simulink model "Z3"  (R2016b)
settings: Solver=VariableStepAuto  StartTime=0.0  StopTime=2  RelTol=1e-3
values from neighbouring files (symbols this model uses):
  x0 = [0.1 0.1 0.1]    [z3.m]    (also in z6.m = [-1 2 1]; z7.m = [0 0 0]; z8.m = [-1 2 1])
settings Model: Creator=E7440  LastModifiedBy=E7440

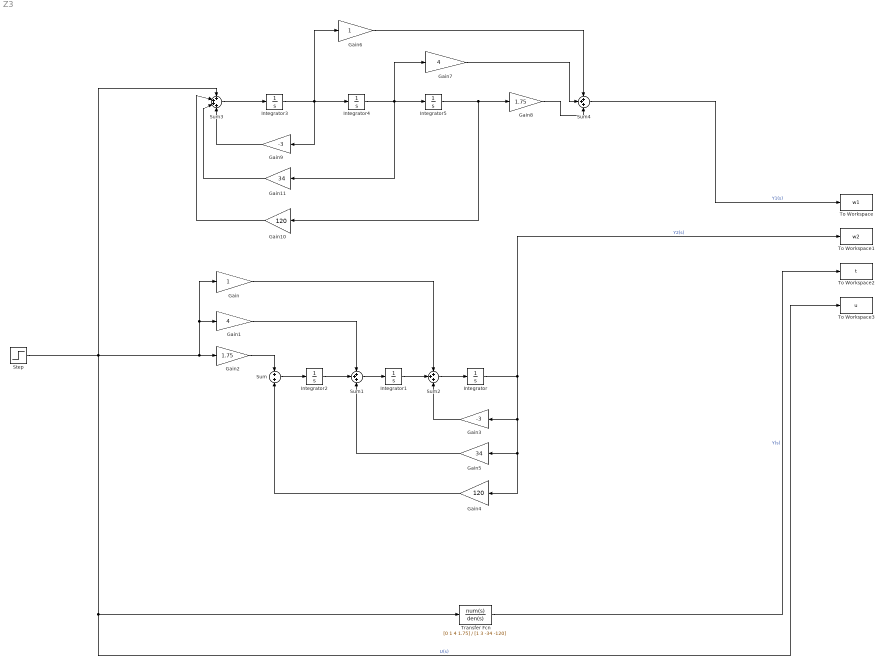
== system Z3 ==
  Gain : Gain
  Gain1 : Gain  Gain=4
  Gain10 : Gain  Gain=120
  Gain11 : Gain  Gain=34
  Gain2 : Gain  Gain=1.75
  Gain3 : Gain  Gain=-3
  Gain4 : Gain  Gain=120
  Gain5 : Gain  Gain=34
  Gain6 : Gain
  Gain7 : Gain  Gain=4
  Gain8 : Gain  Gain=1.75
  Gain9 : Gain  Gain=-3
  Integrator : Integrator  InitialCondition=x0(3)
  Integrator1 : Integrator  InitialCondition=x0(2)
  Integrator2 : Integrator  InitialCondition=x0(1)
  Integrator3 : Integrator  InitialCondition=x0(1)
  Integrator4 : Integrator  InitialCondition=x0(2)
  Integrator5 : Integrator  InitialCondition=x0(3)
  Step : Step  SampleTime=0
  Sum : Sum
  Sum1 : Sum  Inputs=+++
  Sum2 : Sum  Inputs=+++
  Sum3 : Sum  Inputs=++++
  Sum4 : Sum  Inputs=+++
  To Workspace : ToWorkspace  VariableName=w1  SaveFormat=Timeseries  SampleTime=-1
  To Workspace1 : ToWorkspace  VariableName=w2  SaveFormat=Timeseries  SampleTime=-1
  To Workspace2 : ToWorkspace  VariableName=t  SaveFormat=Timeseries  SampleTime=-1
  To Workspace3 : ToWorkspace  VariableName=u  SaveFormat=Timeseries  SampleTime=-1
  Transfer Fcn : TransferFcn  Numerator=[0 1 4 1.75]  Denominator=[1 3 -34 -120]
  wires:
  Sum/1 -> Integrator2/1
  Gain3/1 -> Sum2/3
  Integrator/1 -> To Workspace1/1, Gain3/1, Gain5/1, Gain4/1  "Y2(s)"
  Gain2/1 -> Sum/1
  Integrator1/1 -> Sum2/2
  Sum2/1 -> Integrator/1
  Integrator2/1 -> Sum1/2
  Sum1/1 -> Integrator1/1
  Gain5/1 -> Sum1/3
  Gain4/1 -> Sum/2
  Gain/1 -> Sum2/1
  Gain1/1 -> Sum1/1
  Step/1 -> To Workspace3/1, Transfer Fcn/1, Sum3/1, Gain/1, Gain1/1, Gain2/1  "U(s)"
  Sum3/1 -> Integrator3/1
  Gain8/1 -> Sum4/3
  Gain7/1 -> Sum4/2
  Gain6/1 -> Sum4/1
  Integrator5/1 -> Gain10/1, Gain8/1
  Integrator3/1 -> Integrator4/1, Gain9/1, Gain6/1
  Gain9/1 -> Sum3/4
  Integrator4/1 -> Integrator5/1, Gain11/1, Gain7/1
  Gain10/1 -> Sum3/2
  Gain11/1 -> Sum3/3
  Sum4/1 -> To Workspace/1  "Y1(s)"
  Transfer Fcn/1 -> To Workspace2/1  "Y(s)"
